simulink model "test_xil_est"  (Simulink 6.2)
settings: Solver=ode45  StartTime=0.0  StopTime=10.0  RelTol=1e-3
libraries: xbsIndex_r3 x18
settings Model: LastModifiedBy=mdexter
settings DebuggingCC: SolverPrmCheckMsg=warning

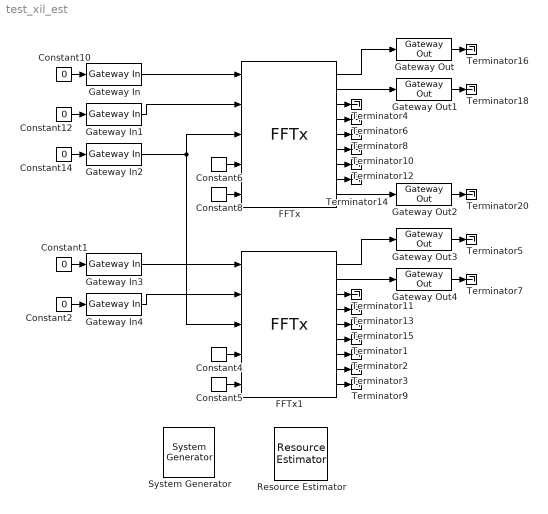
== system test_xil_est ==
  " System Generator" : xbsIndex_r3/ System Generator  Tag=genX  xilinxfamily=Virtex2P  part=xc2vp40  speed=-6  package=ff1152  synthesis_tool=XST  directory=./test_xil_est.netlist  testbench=off  simulink_period=1  sysclk_period=10  incr_netlist=off  trim_vbits=Everywhere in SubSystem  dbl_ovrd=According to Block Masks  core_generation=According to Block Masks  run_coregen=off  deprecated_control=off  eval_field=0
      settings: AttributesFormatString=System\nGenerator
  Constant{1..2,10,12,14} (5 alike) : Constant  Value=0
  Constant{4..6,8} (4 alike) : xbsIndex_r3/Constant  const=1  equ=P=C  arith_type=Boolean  n_bits=1  bin_pt=0  opselect=C  inp2=PCIN>>17  opr=+  inp1=P  carry=CIN  iostate=0  explicit_period=on  period=1  dbl_ovrd=off
  FFTx : xbsIndex_r3/FFTx  arch=Pipelined Streaming I/O  npts=1024  scaling=Unscaled  rounding=Convergent Rounding  tf_width=8  op_order=Bit Reversed Order  twiddle_mem_type=Block RAM  data_mem_type=Block RAM  num_bram_stages=3  explicit_period=off  period=-1  use_dsp48=off  en_n=off  has_ovflo=off  rst=off  en=off  dbl_ovrd=off  show_param=on  gen_core=off
      settings: xl_area=[1040 1163 7 1272 0 6 0]
  FFTx1 : xbsIndex_r3/FFTx  arch=Pipelined Streaming I/O  npts=1024  scaling=Unscaled  rounding=Convergent Rounding  tf_width=8  op_order=Bit Reversed Order  twiddle_mem_type=Block RAM  data_mem_type=Block RAM  num_bram_stages=3  explicit_period=off  period=-1  use_dsp48=off  en_n=off  has_ovflo=off  rst=off  en=off  dbl_ovrd=off  show_param=on  gen_core=off
      settings: xl_area=[1040 1163 7 1272 0 6 0]
  Gateway In{,1,3..4} (4 alike) : xbsIndex_r3/Gateway In  arith_type="Signed  (2's comp)"  n_bits=8  bin_pt=7  quantization=Truncate  overflow=Wrap  period=1  timing_constraint=None  locs_specified=off  LOCs={}  needs_fixed_name=off  dbl_ovrd=off  show_param=off
      settings: xl_area=[0 0 0 0 8 0 0]
  Gateway In2 : xbsIndex_r3/Gateway In  arith_type=Boolean  n_bits=8  bin_pt=7  quantization=Truncate  overflow=Wrap  period=1  timing_constraint=None  locs_specified=off  LOCs={}  needs_fixed_name=off  dbl_ovrd=off  show_param=off
      settings: xl_area=[0 0 0 0 1 0 0]
  Gateway Out{,1..4} (5 alike) : xbsIndex_r3/Gateway Out  output_type=Double  nbits=8  bin_pt=6  arith_type=Boolean  quantization=Truncate  overflow=Wrap  hdl_port=on  timing_constraint=None  locs_specified=off  LOCs={}  needs_fixed_name=off  show_param=off
      Gateway Out settings: xl_area=[0 0 0 0 19 0 0]
      Gateway Out1 settings: xl_area=[0 0 0 0 19 0 0]
      Gateway Out2 settings: xl_area=[0 0 0 0 1 0 0]
      Gateway Out3 settings: xl_area=[0 0 0 0 19 0 0]
      Gateway Out4 settings: xl_area=[0 0 0 0 19 0 0]
  Resource Estimator : xbsIndex_r3/Resource Estimator  Tag=resEstTag  xl_estimator_area=[2080 2326 14 2544 110 12 0]  xl_use_estimator_area=off  simulink_period=1  mrp_directory=./test_xil_est.netlist
      settings: AttributesFormatString=Resource Estimator\n%<xl_estimator_area>\n[SL FF BR LUT IO MUL TBUF]
  Terminator{1..16,18,20} (18 alike) : Terminator
  wires:
  Gateway In1/1 -> FFTx/2
  Constant6/1 -> FFTx/4
  Constant8/1 -> FFTx/5
  FFTx/2 -> Gateway Out1/1
  FFTx/3 -> Terminator4/1
  FFTx/4 -> Terminator6/1
  FFTx/5 -> Terminator8/1
  FFTx/6 -> Terminator10/1
  FFTx/7 -> Terminator12/1
  FFTx/8 -> Terminator14/1
  FFTx/9 -> Gateway Out2/1
  Gateway In/1 -> FFTx/1
  FFTx/1 -> Gateway Out/1
  Gateway In2/1 -> FFTx/3, FFTx1/3
  Constant10/1 -> Gateway In/1
  Constant12/1 -> Gateway In1/1
  Constant14/1 -> Gateway In2/1
  Gateway Out/1 -> Terminator16/1
  Gateway Out1/1 -> Terminator18/1
  Gateway Out2/1 -> Terminator20/1
  Gateway In4/1 -> FFTx1/2
  Constant4/1 -> FFTx1/4
  Constant5/1 -> FFTx1/5
  FFTx1/2 -> Gateway Out4/1
  FFTx1/3 -> Terminator11/1
  FFTx1/4 -> Terminator13/1
  FFTx1/5 -> Terminator15/1
  FFTx1/6 -> Terminator1/1
  FFTx1/7 -> Terminator2/1
  FFTx1/8 -> Terminator3/1
  FFTx1/9 -> Terminator9/1
  Gateway In3/1 -> FFTx1/1
  FFTx1/1 -> Gateway Out3/1
  Constant1/1 -> Gateway In3/1
  Constant2/1 -> Gateway In4/1
  Gateway Out3/1 -> Terminator5/1
  Gateway Out4/1 -> Terminator7/1
